simulink model "DACSimulink"  (R2023a)
settings: Solver=ode23tb  StartTime=0.0  StopTime=TMax  FixedStep=DT  MaxStep=DT  RelTol=1e-3  EnableMultiTasking=on
values from neighbouring files (symbols this model uses):
  A_e = [A_a, Bd_a * H_d; zeros(size(D_d,1),size(A_a,1)), D_d]    [runDACScript.m]
  B_e = [B_a;zeros(size(D_d,1),size(B_a,2))]    [runDACScript.m]
  C_e = [C_a,zeros(size(C_a,1),Ndstates)]    [runDACScript.m]
  K = -[Kx,Kd]    [runDACScript.m]
  OutList = cell(27, 1)    [runDACScript.m]
  PC_MaxPit = 1.570796    [runDACScript.m]
  PC_MaxRat = 0.1396263    [runDACScript.m]
  PC_MinPit = 0.0    (= 0)    [runDACScript.m]
  RE = eye(NOuts)    [runDACScript.m]
  To = 0.3    [runDACScript.m]
undefined symbols (not defined in the file or in its folder): Continuous, strmatch, Time
libraries: ctrlSharedLib x1
settings Model: Creator=jnjiri  LastModifiedBy=Administrator
settings SolverCC: AlgebraicLoopSolver=TrustRegion  SolverResetMethod=Robust
settings DataIOCC: LimitDataPoints=on  SaveFormat=Array  SaveOutput=off  InspectSignalLogs=on  SaveTime=off  ReturnWorkspaceOutputs=off  SignalLoggingName=sigsOut
settings OptimizationCC: ReuseModelBlockBuffer=off  ExpressionDepthLimit=2147483647  LifeSpan=inf
settings DebuggingCC: SaveWithParameterizedLinksMsg=none  UnderspecifiedInitializationDetection=Classic  MergeDetectMultiDrivingBlocksExec=none  SignalResolutionControl=TryResolveAllWithWarning  MultiTaskDSMMsg=warning  MultiTaskCondExecSysMsg=none  UnconnectedInputMsg=warning  UnconnectedOutputMsg=warning  UnconnectedLineMsg=warning  StateNameClashWarn=warning  SFUnexpectedBacktrackingDiag=warning  SFNoUnconditionalDefaultTransitionDiag=warning  SFExecutionAtInitializationDiag=none  ArithmeticOperatorsInVariantConditions=warning
settings HardwareCC: ProdBitPerPointer=32  ProdBitPerSizeT=32  ProdBitPerPtrDiffT=32  ProdLargestAtomicFloat=None  ProdIntDivRoundTo=Undefined  ProdEndianess=Unspecified  ProdWordSize=32  ProdHWDeviceType=32-bit Generic  TargetUnknown=on
settings ModelReferenceCC: EnableRefExpFcnMdlSchedulingChecks=on  PropagateSignalLabelsOutOfModel=off
settings SFSimCC: SimUseLocalCustomCode=off  CustomCodeUndefinedFunction=UseInterfaceOnly
settings RTWCC: RTWUseLocalCustomCode=off
settings CodeAppCC: StateflowObjectComments=on
settings GRTTargetCC: TargetLangStandard=C89/C90 (ANSI)  CombineOutputUpdateFcns=off  GRTInterface=on
settings ConfigComp: CovMetricSettings=dw  CovSaveCumulativeToWorkspaceVar=on  CovSaveSingleToWorkspaceVar=on  CovExternalEMLEnable=off  CovSFcnEnable=off

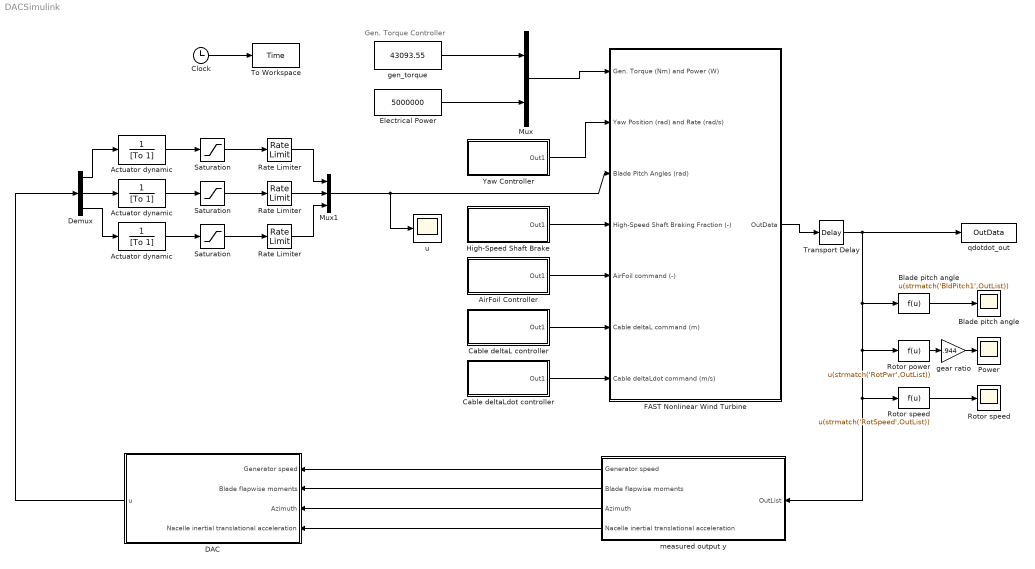
== system DACSimulink ==
  note: Gen. Torque Controller
  " Actuator dynamic " : TransferFcn  Denominator=[To 1]
  " Rate Limiter" : RateLimiter  RisingSlewLimit=PC_MaxRat  FallingSlewLimit=-PC_MaxRat  SampleTimeMode=inherited  LinearizeAsGain=off
  " Rate Limiter " : RateLimiter  RisingSlewLimit=PC_MaxRat  FallingSlewLimit=-PC_MaxRat  SampleTimeMode=inherited  LinearizeAsGain=off
  " Saturation" : Saturate  UpperLimit=PC_MaxPit  LowerLimit=PC_MinPit
  Actuator dynamic : TransferFcn  Denominator=[To 1]
  "Actuator dynamic " : TransferFcn  Denominator=[To 1]
  AirFoil Controller : Subsystem
  Blade pitch angle : Fcn  Expr=u(strmatch('BldPitch1',OutList))
  "Blade pitch angle " : Scope
  Cable deltaL controller : Subsystem
  Cable deltaLdot controller : Subsystem
  Clock : Clock
  DAC : Subsystem
  Demux : Demux  Outputs=3
  Electrical Power : Constant  Value=5000000
  FAST Nonlinear Wind Turbine : Subsystem  mask(FAST Nonlinear Wind Turbine){}
      mask help: This block contains the FAST S-Function.
      mask init:
      | clear FAST_SFunc
  High-Speed Shaft Brake : Subsystem
  Mux : Mux  Inputs=2
  Mux1 : Mux  Inputs=3
  "Power " : Scope
  "Rate Limiter " : RateLimiter  RisingSlewLimit=PC_MaxRat  FallingSlewLimit=-PC_MaxRat  SampleTimeMode=inherited  LinearizeAsGain=off
  Rotor power : Fcn  Expr=u(strmatch('RotPwr',OutList))
  Rotor speed : Fcn  Expr=u(strmatch('RotSpeed',OutList))
  "Rotor speed " : Scope
  "Saturation " : Saturate  UpperLimit=PC_MaxPit  LowerLimit=PC_MinPit
  "Saturation  " : Saturate  UpperLimit=PC_MaxPit  LowerLimit=PC_MinPit
  To Workspace : ToWorkspace  VariableName=Time  SampleTime=-1
  Transport Delay : TransportDelay  DelayTime=0.01
  Yaw Controller : Subsystem
  gear ratio : Gain  Gain=.944
  gen_torque : Constant  Value=43093.55
  measured output y : Subsystem
  qdotdot_out : ToWorkspace  VariableName=OutData  SampleTime=-1
  u : Scope
  wires:
  Clock/1 -> To Workspace/1
  Cable deltaLdot controller/1(Out1) -> FAST Nonlinear Wind Turbine/7(Cable deltaLdot command (m/s))
  High-Speed Shaft Brake/1(Out1) -> FAST Nonlinear Wind Turbine/4(High-Speed Shaft Braking Fraction (-))
  AirFoil Controller/1(Out1) -> FAST Nonlinear Wind Turbine/5(AirFoil command (-))
  Cable deltaL controller/1(Out1) -> FAST Nonlinear Wind Turbine/6(Cable deltaL command (m))
  Mux/1 -> FAST Nonlinear Wind Turbine/1(Gen. Torque (Nm) and Power (W))
  Yaw Controller/1(Out1) -> FAST Nonlinear Wind Turbine/2(Yaw Position (rad) and Rate (rad/s))
  FAST Nonlinear Wind Turbine/1(OutData) -> Transport Delay/1
  Mux1/1 -> u/1, FAST Nonlinear Wind Turbine/3(Blade Pitch Angles (rad))
  Blade pitch angle/1 -> "Blade pitch angle "/1
  Demux/3 -> " Actuator dynamic "/1
  " Actuator dynamic "/1 -> " Saturation"/1
  Demux/2 -> Actuator dynamic/1
  Actuator dynamic/1 -> "Saturation  "/1
  Demux/1 -> "Actuator dynamic "/1
  "Actuator dynamic "/1 -> "Saturation "/1
  " Rate Limiter"/1 -> Mux1/1
  DAC/1(u) -> Demux/1
  " Rate Limiter "/1 -> Mux1/2
  "Rate Limiter "/1 -> Mux1/3
  " Saturation"/1 -> "Rate Limiter "/1
  "Saturation  "/1 -> " Rate Limiter "/1
  "Saturation "/1 -> " Rate Limiter"/1
  measured output y/4("Nacelle inertial translational acceleration ") -> DAC/4("Nacelle inertial translational acceleration ")
  measured output y/1("Generator speed ") -> DAC/1(Generator speed)
  Transport Delay/1 -> measured output y/1(OutList), Rotor speed/1, Rotor power/1, Blade pitch angle/1, qdotdot_out/1
  measured output y/3(Azimuth) -> DAC/3(Azimuth)
  measured output y/2(Blade flapwise moments) -> DAC/2(Blade flapwise moments)
  gen_torque/1 -> Mux/1
  Electrical Power/1 -> Mux/2
  Rotor speed/1 -> "Rotor speed "/1
  Rotor power/1 -> gear ratio/1
  gear ratio/1 -> "Power "/1

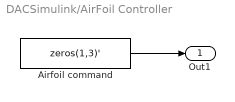
== system DACSimulink/AirFoil Controller ==
  Airfoil command : Constant  Value=zeros(1,3)'
  Out1 : Outport
  wires:
  Airfoil command/1 -> Out1/1

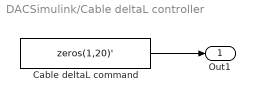
== system DACSimulink/Cable deltaL controller ==
  Cable deltaL command : Constant  Value=zeros(1,20)'
  Out1 : Outport
  wires:
  Cable deltaL command/1 -> Out1/1

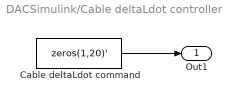
== system DACSimulink/Cable deltaLdot controller ==
  Cable deltaLdot command : Constant  Value=zeros(1,20)'
  Out1 : Outport
  wires:
  Cable deltaLdot command/1 -> Out1/1

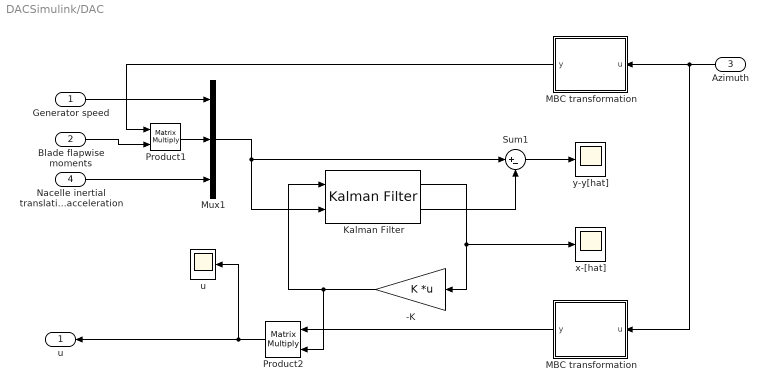
== system DACSimulink/DAC ==
  Generator speed : Inport
  Blade flapwise moments : Inport  Port=2
  Azimuth : Inport  Port=3
  "Nacelle inertial translational acceleration " : Inport  Port=4
  -K : Gain  Gain=K  Multiplication=Matrix(K*u)
  "Kalman Filter " : ctrlSharedLib/Kalman Filter  TimeDomain=Continuous-Time  UseCurrentEstimator=on  ModelSource=Individual A, B, C, D matrices  ModelSourceVariable=ss(0.95,1,1,0,1)  A=A_e  B=B_e  C=C_e  D=0  NumberOfStates=1  NumberOfInputs=1  NumberOfOutputs=1  InitialEstimateSource=Dialog  X0=0  P0=10  UseK=off  UseGH=off  NumberOfProcessNoiseInputs=1  G=1  TimeInvariantG=on  H=0  TimeInvariantH=on  Q=QE  TimeInvariantQ=on  R=RE  TimeInvariantR=on  N=0  TimeInvariantN=on  AddInputPort=on  AddEnablePort=off  OutputEstimatedY=on  OutputP=off  Ts=-1
  MBC transformation : MATLAB Function  TreatAsAtomicUnit=on
  "MBC transformation " : MATLAB Function  TreatAsAtomicUnit=on
  Mux1 : Mux  Inputs=3
  Product1 : Product  Multiplication=Matrix(*)
  Product2 : Product  Multiplication=Matrix(*)
  Sum1 : Sum  Inputs=|+-
  "u " : Scope
  x-[hat] : Scope
  y-y[hat] : Scope
  u : Outport
  wires:
  "Kalman Filter "/1 -> -K/1, x-[hat]/1
  Azimuth/1 -> MBC transformation/1(u), "MBC transformation "/1(u)
  Blade flapwise moments/1 -> Product1/2
  "MBC transformation "/1(y) -> Product1/1
  -K/1 -> Product2/2, "Kalman Filter "/1
  MBC transformation/1(y) -> Product2/1
  Mux1/1 -> "Kalman Filter "/2, Sum1/1
  Generator speed/1 -> Mux1/1
  "Nacelle inertial translational acceleration "/1 -> Mux1/3
  "Kalman Filter "/2 -> Sum1/2
  Sum1/1 -> y-y[hat]/1
  Product1/1 -> Mux1/2
  Product2/1 -> u/1, "u "/1

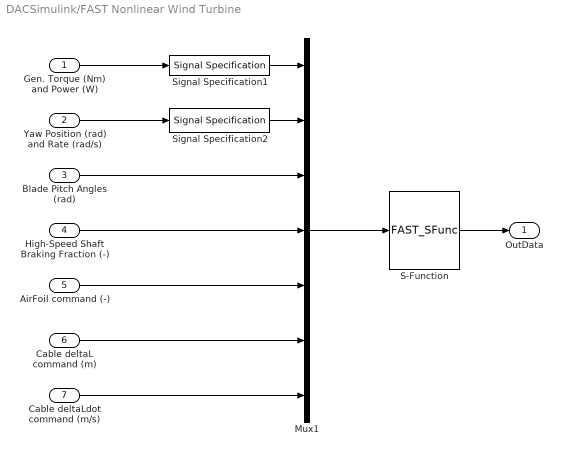
== system DACSimulink/FAST Nonlinear Wind Turbine ==
  Gen. Torque (Nm) and Power (W) : Inport
  Yaw Position (rad) and Rate (rad/s) : Inport  Port=2
  Blade Pitch Angles (rad) : Inport  Port=3
  High-Speed Shaft Braking Fraction (-) : Inport  Port=4
  AirFoil command (-) : Inport  Port=5
  Cable deltaL command (m) : Inport  Port=6
  Cable deltaLdot command (m/s) : Inport  Port=7
  Mux1 : Mux  Inputs=7
  S-Function : S-Function  FunctionName=FAST_SFunc  Parameters=FAST_InputFileName, TMax, 0  SFunctionDeploymentMode=off  EnableBusSupport=off
  Signal Specification1 : SignalSpecification  OutDataTypeStr=double  Dimensions=2
  Signal Specification2 : SignalSpecification  OutDataTypeStr=double  Dimensions=2
  OutData : Outport
  wires:
  Gen. Torque (Nm) and Power (W)/1 -> Signal Specification1/1
  S-Function/1 -> OutData/1
  Mux1/1 -> S-Function/1
  Blade Pitch Angles (rad)/1 -> Mux1/3
  Yaw Position (rad) and Rate (rad/s)/1 -> Signal Specification2/1
  Signal Specification1/1 -> Mux1/1
  Signal Specification2/1 -> Mux1/2
  High-Speed Shaft Braking Fraction (-)/1 -> Mux1/4
  AirFoil command (-)/1 -> Mux1/5
  Cable deltaL command (m)/1 -> Mux1/6
  Cable deltaLdot command (m/s)/1 -> Mux1/7

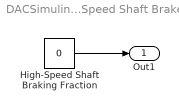
== system DACSimulink/High-Speed Shaft Brake ==
  High-Speed Shaft Braking Fraction : Constant  Value=0
  Out1 : Outport
  wires:
  High-Speed Shaft Braking Fraction/1 -> Out1/1

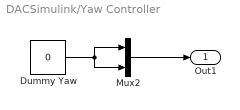
== system DACSimulink/Yaw Controller ==
  Dummy Yaw : Constant  Value=0
  Mux2 : Mux  Inputs=2
  Out1 : Outport
  wires:
  Mux2/1 -> Out1/1
  Dummy Yaw/1 -> Mux2/2, Mux2/1

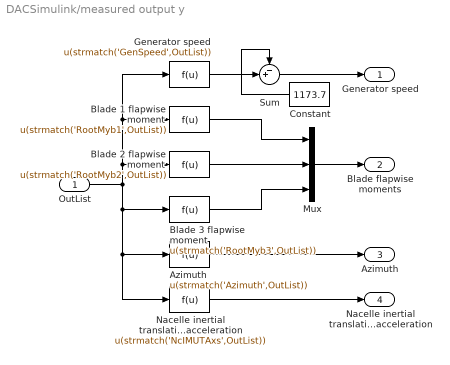
== system DACSimulink/measured output y ==
  OutList : Inport
  "Azimuth " : Fcn  Expr=u(strmatch('Azimuth',OutList))
  Blade 1 flapwise moment : Fcn  Expr=u(strmatch('RootMyb1',OutList))
  Blade 2 flapwise moment : Fcn  Expr=u(strmatch('RootMyb2',OutList))
  Blade 3 flapwise moment : Fcn  Expr=u(strmatch('RootMyb3',OutList))
  Constant : Constant  Value=1173.7
  Generator speed : Fcn  Expr=u(strmatch('GenSpeed',OutList))
  Mux : Mux  Inputs=3
  Nacelle inertial translational acceleration : Fcn  Expr=u(strmatch('NcIMUTAxs',OutList))
  Sum : Sum  Inputs=-+|
  "Generator speed " : Outport
  Blade flapwise moments : Outport  Port=2
  Azimuth : Outport  Port=3
  "Nacelle inertial translational acceleration " : Outport  Port=4
  wires:
  Mux/1 -> Blade flapwise moments/1
  "Azimuth "/1 -> Azimuth/1
  Nacelle inertial translational acceleration/1 -> "Nacelle inertial translational acceleration "/1
  OutList/1 -> Generator speed/1, Blade 1 flapwise moment/1, Blade 2 flapwise moment/1, Nacelle inertial translational acceleration/1, "Azimuth "/1, Blade 3 flapwise moment/1
  Sum/1 -> "Generator speed "/1
  Blade 1 flapwise moment/1 -> Mux/1
  Blade 2 flapwise moment/1 -> Mux/2
  Blade 3 flapwise moment/1 -> Mux/3
  Generator speed/1 -> Sum/2
  Constant/1 -> Sum/1

== matlab function DACSimulink/DAC/MBC transformation ==
  data: u input; y output
function y = fcn(u)
%#codegen
u=(u*pi/180);
y =[1 cos(u) sin(u);1 cos(u+(2*pi/3)) sin(u+(2*pi/3));1 cos(u+(4*pi/3)) sin(u+(4*pi/3))];

== matlab function DACSimulink/DAC/MBC transformation  ==
  data: u input; y output
function y = fcn(u)
%#codegen
u=(u*pi/180);
y =[1/3 1/3 1/3; (2/3)*cos(u) (2/3)*cos(u+(2*pi/3)) (2/3)*cos(u+(4*pi/3)); (2/3)*sin(u) (2/3)*sin(u+(2*pi/3)) (2/3)*sin(u+(4*pi/3))];
